simulink model "v"  (R2016b)
settings: Solver=VariableStepAuto  StartTime=0.0  StopTime=10.0  RelTol=1e-3
settings Model: Creator=Tao  LastModifiedBy=Administrator

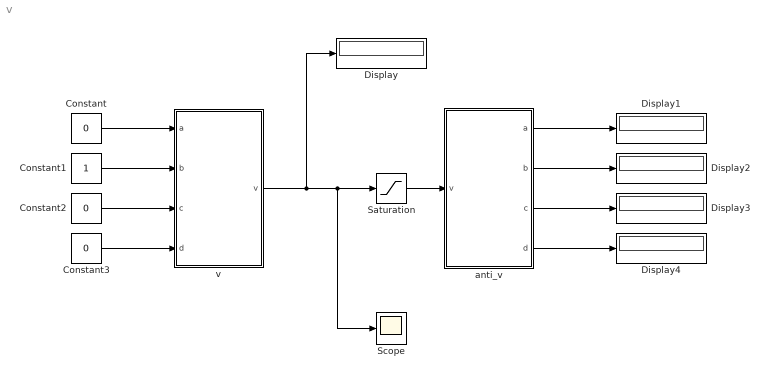
== system v ==
  Constant : Constant  Value=0
  Constant1 : Constant
  Constant2 : Constant  Value=0
  Constant3 : Constant  Value=0
  Display{,1..4} (5 alike) : Display
  Saturation : Saturate  UpperLimit=2147483647  LowerLimit=-2147483647
  Scope : Scope
  anti_v : MATLAB Function  TreatAsAtomicUnit=on
  v : MATLAB Function  TreatAsAtomicUnit=on
  wires:
  Constant3/1 -> v/4(d)
  Constant2/1 -> v/3(c)
  Constant1/1 -> v/2(b)
  Constant/1 -> v/1(a)
  v/1(v) -> Scope/1, Saturation/1, Display/1
  anti_v/1(a) -> Display1/1
  anti_v/4(d) -> Display4/1
  anti_v/3(c) -> Display3/1
  anti_v/2(b) -> Display2/1
  Saturation/1 -> anti_v/1(v)

== matlab function v/anti_v ==
  data: v input; a output; b output; c output; d output
function [a, b, c, d]  = anti_velocity(v)
if v>=0
    BASE = '00000000000000000000000000000000';%一共32位
    Vbin = dec2bin(v);
    LVbin = length(Vbin);
    for i = 1:LVbin
        BASE(32-LVbin+i) = Vbin(i);
    end
    Vbin = BASE;
else
    BASE = '00000000000000000000000000000000';%一共32位
    V = 4294967295 + v + 1; %bin2dec('11111111111111111111111111111111')（一共32位）=4294967295
    Vbin = dec2bin(V);
    LVbin = length(Vbin);
    for i = 1:LVbin
        BASE(32-LVbin+i) = Vbin(i);
    end
    Vbin = BASE;
end
D = Vbin(1:8);
C = Vbin(9:16);
B = Vbin(17:24);
A = Vbin(25:32);
d = bin2dec(D);
c = bin2dec(C);
b = bin2dec(B);
a = bin2dec(A);
end

== matlab function v/v ==
  data: a input; v output; b input; c input; d input
function v  = velocity(a, b, c, d)
A = dec2bin(a);
B = dec2bin(b);
C = dec2bin(c);
D = dec2bin(d);

BASE = '00000000';
LA = length(A);
for i = 1:LA
    BASE(8-LA+i) = A(i);
end
A = BASE;

BASE = '00000000';
LB = length(B);
for i = 1:LB
    BASE(8-LB+i) = B(i);
end
B = BASE;

BASE = '00000000';
LC = length(C);
for i = 1:LC
    BASE(8-LC+i) = C(i);
end
C = BASE;

BASE = '00000000';
LD = length(D);
for i = 1:LD
    BASE(8-LD+i) = D(i);
end
D = BASE;

Vbin = [D, C, B, A];
V = bin2dec(Vbin);
if d < 128  %bin2dec('10000000')=128
    v = V;
else
    V = V-1;
    v = -(4294967295 - V); %bin2dec('11111111111111111111111111111111')（一共32位）=4294967295
end
